simulink model "SelfLoop"  (R2020b)
settings: Solver=VariableStepAuto  StartTime=0.0  StopTime=10.0  RelTol=1e-3
settings Model: Creator=apple  LastModifiedBy=apple

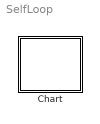
== system SelfLoop ==
  Chart : Stateflow chart  TreatAsAtomicUnit=on

== stateflow chart SelfLoop/Chart ==
  state A
    en:fprintf("Entry A");
    du:fprintf("During A");
    ex:fprintf("Exit A");
  state B
    en:fprintf("Entry B");
    du:fprintf("During B");
    ex:fprintf("Exit B");
  (default) -> A : {x = 0;}
  (junction 3) -> A [order 2] : /{x = x + 1;}
  A -> (junction 3) : E_one
  (junction 3) -> B [order 1] : [x > 3]/{fprintf("Transition Action1");}
  data: x local
  events: E_one local FUNCTION_CALL_EVENT
